simulink model "OperationalSpaceInverseDynamic"  (R2020a)
settings: Solver=VariableStepAuto  StartTime=0.0  StopTime=2.0  RelTol=1e-3
values from neighbouring files (symbols this model uses):
  g = 9.81    [params.m]
  KD = 2*z*w    [params.m]
  KP = w^2    [params.m]
  traj_on = 1    [params.m]
libraries: simulink x1, robotcorelib x1, vrlib x1
settings Model: Creator=Sebastiano  LastModifiedBy=Sebastiano

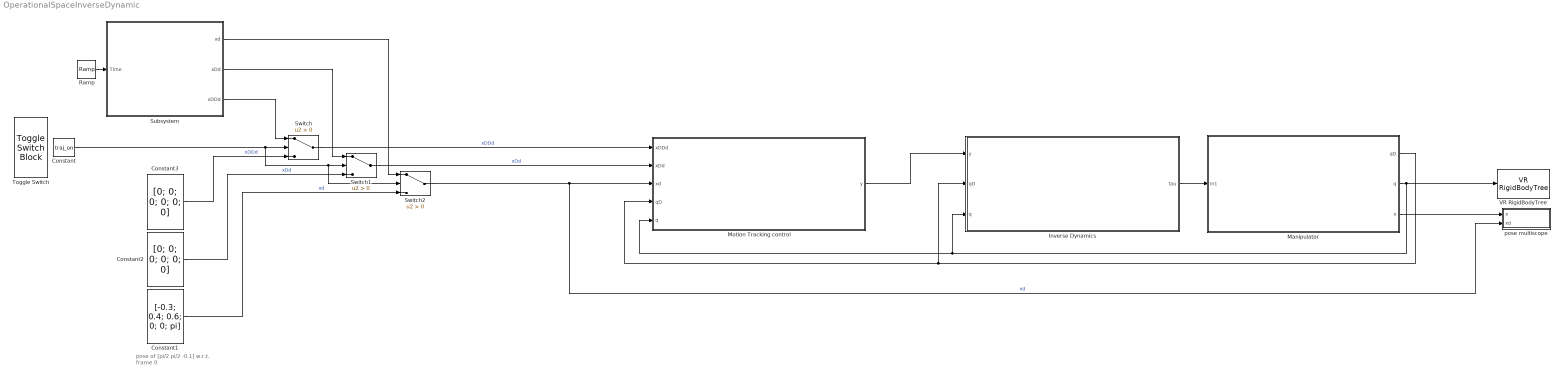
== system OperationalSpaceInverseDynamic ==
  note: pose of [pi/2 pi/2 -0.1]
      | w.r.t. frame 0
  Constant : Constant  Value=traj_on
  Constant1 : Constant  Value=[-0.3; 0.4; 0.6; 0; 0; pi]  VectorParams1D=off
  Constant2 : Constant  Value=[0; 0; 0; 0; 0; 0]  VectorParams1D=off
  Constant3 : Constant  Value=[0; 0; 0; 0; 0; 0]  VectorParams1D=off
  Inverse Dynamics : Subsystem
  Manipulator : Subsystem
  Motion Tracking control : Subsystem
  Ramp : simulink/Sources/Ramp  slope=1  start=0  InitialOutput=0
  Subsystem : Subsystem
  Switch : Switch  Criteria=u2 > Threshold
  Switch1 : Switch  Criteria=u2 > Threshold
  Switch2 : Switch  Criteria=u2 > Threshold
  Toggle Switch : ToggleSwitchBlock  LabelPosition=Hide
      settings: Values={{'Steady-State', 'Trajectory'}, [0 1]}
  VR RigidBodyTree : vrlib/VR RigidBodyTree  RBT=robot  useRBT=on  Ts=-1  ForceViewerOpen=on
      settings: SourceProductBaseCode=SL
  pose multiscope : Subsystem
  wires:
  Switch2/1 -> pose multiscope/2(xd), Motion Tracking control/3(xd)  "xd"
  Switch/1 -> Motion Tracking control/1(xDDd)  "xDDd"
  Switch1/1 -> Motion Tracking control/2(xDd)  "xDd"
  Manipulator/1(qD) -> Inverse Dynamics/2(qD), Motion Tracking control/4(qD)
  Manipulator/2(q) -> Motion Tracking control/5(q), Inverse Dynamics/3(q), VR RigidBodyTree/1
  Inverse Dynamics/1(tau) -> Manipulator/1(In1)
  Motion Tracking control/1(y) -> Inverse Dynamics/1(y)
  Manipulator/3(x) -> pose multiscope/1(x)
  Constant2/1 -> Switch1/3  "xDd"
  Constant/1 -> Switch2/2, Switch1/2, Switch/2
  Constant1/1 -> Switch2/3  "xd"
  Constant3/1 -> Switch/3  "xDDd"
  Ramp/1 -> Subsystem/1(Time)
  Subsystem/3(xDDd) -> Switch/1
  Subsystem/2(xDd) -> Switch1/1
  Subsystem/1(xd) -> Switch2/1

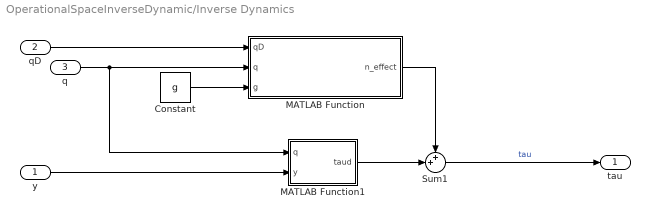
== system OperationalSpaceInverseDynamic/Inverse Dynamics ==
  y : Inport
  qD : Inport  Port=2
  q : Inport  Port=3
  Constant : Constant  Value=g
  MATLAB Function : MATLAB Function  TreatAsAtomicUnit=on
  MATLAB Function1 : MATLAB Function  TreatAsAtomicUnit=on
  Sum1 : Sum  Inputs=++|
  tau : Outport
  wires:
  qD/1 -> MATLAB Function/1(qD)
  MATLAB Function/1(n_effect) -> Sum1/1
  MATLAB Function1/1(taud) -> Sum1/2
  q/1 -> MATLAB Function/2(q), MATLAB Function1/1(q)
  Constant/1 -> MATLAB Function/3(g)
  y/1 -> MATLAB Function1/2(y)
  Sum1/1 -> tau/1  "tau"

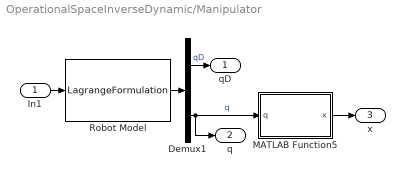
== system OperationalSpaceInverseDynamic/Manipulator ==
  In1 : Inport
  Demux1 : Demux  Outputs=[3, 3]
  MATLAB Function5 : MATLAB Function  TreatAsAtomicUnit=on
  Robot Model : S-Function  FunctionName=LagrangeFormulation  Parameters=g  SFunctionDeploymentMode=off  EnableBusSupport=off
  qD : Outport
  q : Outport  Port=2
  x : Outport  Port=3
  wires:
  In1/1 -> Robot Model/1
  Robot Model/1 -> Demux1/1
  Demux1/2 -> MATLAB Function5/1(q), q/1  "q"
  Demux1/1 -> qD/1  "qD"
  MATLAB Function5/1(x) -> x/1

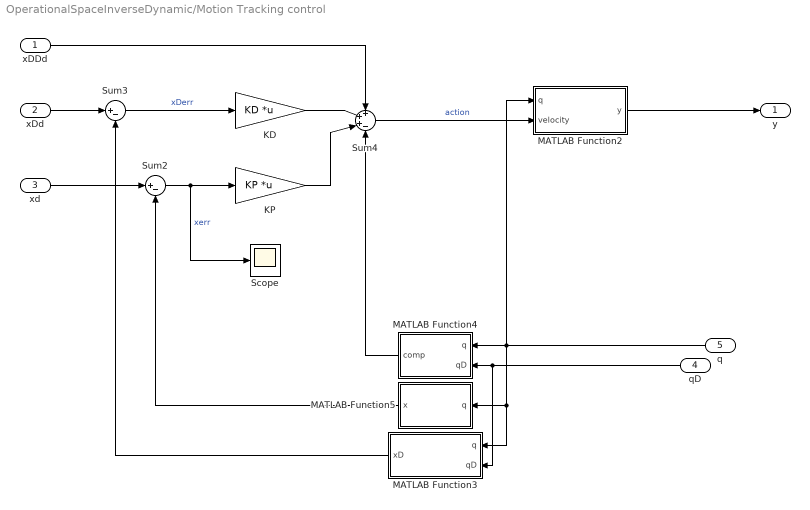
== system OperationalSpaceInverseDynamic/Motion Tracking control ==
  xDDd : Inport
  xDd : Inport  Port=2
  xd : Inport  Port=3
  qD : Inport  Port=4
  q : Inport  Port=5
  KD : Gain  Gain=KD  Multiplication=Matrix(K*u) (u vector)
  KP : Gain  Gain=KP  Multiplication=Matrix(K*u) (u vector)
  MATLAB Function2 : MATLAB Function  TreatAsAtomicUnit=on
  MATLAB Function3 : MATLAB Function  TreatAsAtomicUnit=on
  MATLAB Function4 : MATLAB Function  TreatAsAtomicUnit=on
  MATLAB Function5 : MATLAB Function  TreatAsAtomicUnit=on
  Scope : Scope
  Sum2 : Sum  Inputs=|+-
  Sum3 : Sum  Inputs=|+-
  Sum4 : Sum  Inputs=+++-
  y : Outport
  wires:
  MATLAB Function2/1(y) -> y/1
  xDd/1 -> Sum3/1
  xDDd/1 -> Sum4/1
  xd/1 -> Sum2/1
  MATLAB Function3/1(xD) -> Sum3/2
  KP/1 -> Sum4/3
  Sum4/1 -> MATLAB Function2/2(velocity)  "action"
  qD/1 -> MATLAB Function3/2(qD), MATLAB Function4/2(qD)
  q/1 -> MATLAB Function3/1(q), MATLAB Function5/1(q), MATLAB Function4/1(q), MATLAB Function2/1(q)
  Sum3/1 -> KD/1  "xDerr"
  MATLAB Function5/1(x) -> Sum2/2
  MATLAB Function4/1(comp) -> Sum4/4
  Sum2/1 -> KP/1, Scope/1  "xerr"
  KD/1 -> Sum4/2

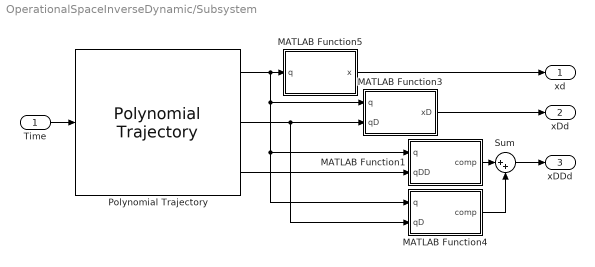
== system OperationalSpaceInverseDynamic/Subsystem ==
  Time : Inport
  MATLAB Function1 : MATLAB Function  TreatAsAtomicUnit=on
  MATLAB Function3 : MATLAB Function  TreatAsAtomicUnit=on
  MATLAB Function4 : MATLAB Function  TreatAsAtomicUnit=on
  MATLAB Function5 : MATLAB Function  TreatAsAtomicUnit=on
  Polynomial Trajectory : robotcorelib/Polynomial Trajectory  WaypointSource=Internal  Waypoints=[ pi/4, -pi/2, pi/4; -pi/4, pi/4, -pi/6; 0.1, -0.1, 0.2]  TimePoints=[ 0, 1.5, 2 ]  TimeInterval=[ 1, 4 ]  Method=Cubic Polynomial  ParameterSource=Internal  VelocityBoundaryCondition=zeros( 3, 3 )  AccelerationBoundaryCondition=zeros( 2, 5 )  SimulateUsing=Interpreted execution
      settings: SourceProductBaseCode=NV,RO,RR
  Sum : Sum  Inputs=|++
  xd : Outport
  xDd : Outport  Port=2
  xDDd : Outport  Port=3
  wires:
  Sum/1 -> xDDd/1
  Polynomial Trajectory/1 -> MATLAB Function3/1(q), MATLAB Function4/1(q), MATLAB Function1/1(q), MATLAB Function5/1(q)
  MATLAB Function4/1(comp) -> Sum/2
  MATLAB Function3/1(xD) -> xDd/1
  Polynomial Trajectory/2 -> MATLAB Function3/2(qD), MATLAB Function4/2(qD)
  MATLAB Function1/1(comp) -> Sum/1
  Polynomial Trajectory/3 -> MATLAB Function1/2(qDD)
  Time/1 -> Polynomial Trajectory/1
  MATLAB Function5/1(x) -> xd/1

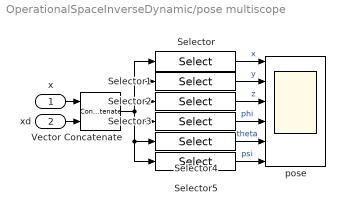
== system OperationalSpaceInverseDynamic/pose multiscope ==
  x : Inport
  xd : Inport  Port=2
  Selector : Selector  NumberOfDimensions=2  InputPortWidth=3  IndexOptions=Index vector (dialog),Select all  Indices=1,7  OutputSizes=6,6
  Selector1 : Selector  NumberOfDimensions=2  InputPortWidth=3  IndexOptions=Index vector (dialog),Select all  Indices=2,7  OutputSizes=6,6
  Selector2 : Selector  NumberOfDimensions=2  InputPortWidth=3  IndexOptions=Index vector (dialog),Select all  Indices=3,7  OutputSizes=6,6
  Selector3 : Selector  NumberOfDimensions=2  InputPortWidth=3  IndexOptions=Index vector (dialog),Select all  Indices=4,7  OutputSizes=6,6
  Selector4 : Selector  NumberOfDimensions=2  InputPortWidth=3  IndexOptions=Index vector (dialog),Select all  Indices=5,7  OutputSizes=6,6
  Selector5 : Selector  NumberOfDimensions=2  InputPortWidth=3  IndexOptions=Index vector (dialog),Select all  Indices=6,7  OutputSizes=6,6
  Vector Concatenate : Concatenate  Mode=Multidimensional array  ConcatenateDimension=2
  pose : Scope  NumInputPorts=6
  wires:
  x/1 -> Vector Concatenate/1
  xd/1 -> Vector Concatenate/2
  Selector1/1 -> pose/2  "y"
  Selector5/1 -> pose/6  "psi"
  Selector3/1 -> pose/4  "phi"
  Selector/1 -> pose/1  "x"
  Selector4/1 -> pose/5  "theta"
  Vector Concatenate/1 -> Selector/1, Selector1/1, Selector2/1, Selector5/1, Selector4/1, Selector3/1
  Selector2/1 -> pose/3  "z"

== matlab function OperationalSpaceInverseDynamic/Subsystem/MATLAB Function3 ==
  data: q input; xD output; qD input
function xD = JA(q, qD)

xD = AnalyticalJacobian(q)*qD;

== matlab function OperationalSpaceInverseDynamic/Motion Tracking control/MATLAB Function2 ==
  data: q input; y output; velocity input
function y = JAinv(q, velocity)

y = pinv(AnalyticalJacobian(q)) * velocity;

== matlab function OperationalSpaceInverseDynamic/Motion Tracking control/MATLAB Function3 ==
  data: q input; xD output; qD input
function xD = JA(q, qD)

xD = AnalyticalJacobian(q)*qD;

== matlab function OperationalSpaceInverseDynamic/Motion Tracking control/MATLAB Function4 ==
  data: q input; comp output; qD input
function comp = JAD(q, qD)

t1 = q(1);
t2 = q(2);
d3 = q(3);

Dt1 = qD(1);
Dt2 = qD(2);
Dd3 = qD(3);

JAD = [[ - 2/5*Dt1*cos(t1) - 3/10*cos(t1 + t2)*(Dt1 + Dt2), -3/10*cos(t1 + t2)*(Dt1 + Dt2), 0];
       [ - 3/10*sin(t1 + t2)*(Dt1 + Dt2) - 2/5*Dt1*sin(t1), -3/10*sin(t1 + t2)*(Dt1 + Dt2), 0];
       [                                                 0,                              0, 0];
       [                                                 0,                              0, 0];
       [                                                 0,                              0, 0];
       [                                                 0,                              0, 0]];

comp = JAD*qD;

== matlab function OperationalSpaceInverseDynamic/Motion Tracking control/MATLAB Function5 ==
  data: q input; x output
function x = K(q)

t1 = q(1);
t2 = q(2);
d3 = q(3);

K = [[ cos(t1 + t2), -sin(t1 + t2), 0, (3*cos(t1 + t2))/10 + (2*cos(t1))/5]
     [ sin(t1 + t2),  cos(t1 + t2), 0, (3*sin(t1 + t2))/10 + (2*sin(t1))/5]
     [            0,             0, 1,                            d3 + 2/5]
     [            0,             0, 0,                                   1]];

pos = K(1:3, 4);
ori = rotm2eul(K(1:3,1:3), 'ZYZ')';

x = [pos; ori];

== matlab function OperationalSpaceInverseDynamic/Inverse Dynamics/MATLAB Function ==
  data: qD input; q input; n_effect output; g input
function n_effect = n(qD, q, g)

n_effect = C_Lagrangian(q, qD)*qD + G_Lagrangian(q, g);

== matlab function OperationalSpaceInverseDynamic/Inverse Dynamics/MATLAB Function1 ==
  data: q input; taud output; y input
function taud = B(q, y)

taud = B_Lagrangian(q)*y;

== matlab function OperationalSpaceInverseDynamic/Subsystem/MATLAB Function4 ==
  data: q input; comp output; qD input
function comp = JAD(q, qD)

t1 = q(1);
t2 = q(2);
d3 = q(3);

Dt1 = qD(1);
Dt2 = qD(2);
Dd3 = qD(3);

JAD = [[ - 2/5*Dt1*cos(t1) - 3/10*cos(t1 + t2)*(Dt1 + Dt2), -3/10*cos(t1 + t2)*(Dt1 + Dt2), 0];
       [ - 3/10*sin(t1 + t2)*(Dt1 + Dt2) - 2/5*Dt1*sin(t1), -3/10*sin(t1 + t2)*(Dt1 + Dt2), 0];
       [                                                 0,                              0, 0];
       [                                                 0,                              0, 0];
       [                                                 0,                              0, 0];
       [                                                 0,                              0, 0]];

comp = JAD*qD;

== matlab function OperationalSpaceInverseDynamic/Subsystem/MATLAB Function5 ==
  data: q input; x output
function x = K(q)

t1 = q(1);
t2 = q(2);
d3 = q(3);

K = [[ cos(t1 + t2), -sin(t1 + t2), 0, (3*cos(t1 + t2))/10 + (2*cos(t1))/5]
     [ sin(t1 + t2),  cos(t1 + t2), 0, (3*sin(t1 + t2))/10 + (2*sin(t1))/5]
     [            0,             0, 1,                            d3 + 2/5]
     [            0,             0, 0,                                   1]];

pos = K(1:3, 4);
ori = rotm2eul(K(1:3,1:3), 'ZYZ')';

x = [pos; ori];

== matlab function OperationalSpaceInverseDynamic/Subsystem/MATLAB Function1 ==
  data: q input; comp output; qDD input
function comp = JA(q, qDD)

comp = AnalyticalJacobian(q)*qDD;

== matlab function OperationalSpaceInverseDynamic/Manipulator/MATLAB Function5 ==
  data: q input; x output
function x = K(q)

t1 = q(1);
t2 = q(2);
d3 = q(3);

K = [[ cos(t1 + t2), -sin(t1 + t2), 0, (3*cos(t1 + t2))/10 + (2*cos(t1))/5]
     [ sin(t1 + t2),  cos(t1 + t2), 0, (3*sin(t1 + t2))/10 + (2*sin(t1))/5]
     [            0,             0, 1,                            d3 + 2/5]
     [            0,             0, 0,                                   1]];

pos = K(1:3, 4);
ori = rotm2eul(K(1:3,1:3), 'ZYZ')';

x = [pos; ori];
